simulink model "HEasy"  (Simulink 7.9)
settings: Solver=FixedStepDiscrete  StartTime=0.0  StopTime=1000000000.0  FixedStep=1  RelTol=1e-3
settings Model: Creator=boakes  LastModifiedBy=boakes
settings OptimizationCC: InlineParams=on  InlineInvariantSignals=on  EnhancedBackFolding=on
settings RTWCC: GenCodeOnly=on

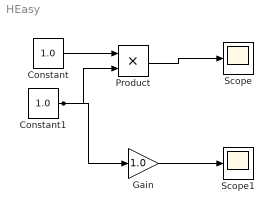
== system HEasy ==
  Constant : Constant  Value=1.0
  Constant1 : Constant  Value=1.0
  Gain : Gain  Gain=1.0
  Product : Product  RndMeth=Zero
  Scope : Scope
      settings: SaveName=ScopeData2
  Scope1 : Scope
      settings: SaveName=ScopeData2
  wires:
  Product/1 -> Scope/1
  Constant/1 -> Product/1
  Gain/1 -> Scope1/1
  Constant1/1 -> Gain/1, Product/2
